simulink model "Cruise_Model_V12_CheckLin_MF"  (R2024a)
settings: Solver=VariableStepAuto  StartTime=0.0  StopTime=0.4  RelTol=1e-9
values from neighbouring files (symbols this model uses):
  coefficients =     [alexisignoringme3.mat]    (also in alexisignoringme4.mat)
  referenceGeo =     [alexisignoringme2.mat]    (also in alexisignoringme3.mat; alexisignoringme4.mat)
  sys = sysMat{i}    [createGainMat.m]    (also in testGains.m = sysMat{idx})
  Ue = [0.0166337400043 -5.79889018864e-09 -1.23056551726e-07 67.3559587388 0 1.57079632679 0 67.3557646602 0 1.57079632679 0 67.3619105721 ... (19 elements, 19x1)]    [alexisignoringme2.mat]    (also in alexisignoringme3.mat = [0.01662518914 6.61806403433e-08 9.21309449136e-07 1460.2523; alexisignoringme4.mat = [0 0 0 0 0 -1471.90874183 1.06985703496e-06 -4.11944256484e-; plotLQI_LQR_Comparison.m = Ut(:,idx(i)+1); testGains.m = U(:,idx+1))
  uref = [0.0193376442889 1.48757714448e-07 3.9703360685e-06 34.4337400406 0 1.41812999309 0 34.4385558366 0 1.41812999309 0 34.4274755705 ... (19 elements, 19x1)]    [alexisignoringme2.mat]    (also in alexisignoringme3.mat; alexisignoringme4.mat)
  Xe = [24.9700402552 0 -1.16861141766 0 0 0 1.12298779449e-07 -0.0450942805758 0.321650208764]    [alexisignoringme2.mat]    (also in alexisignoringme3.mat = [24.9726490597 0 -1.16896704065 0 0 0 -8.24889531393e-07 -0.; alexisignoringme4.mat = [24.9726490597 0 -1.16896704065 0 0 0 -8.24889531393e-07 0.0; plotLQI_LQR_Comparison.m = X(:,idx(i)+1); testGains.m = X(:,idx+1))
  Xes = [24.97004028 0 -1.16861086303 0 0 0 -5.01724449102e-07 -0.0450956248882 0.321650295301]    [alexisignoringme2.mat]    (also in alexisignoringme3.mat = [0.00351658839646 0 -9.99999599468 0 0 0 2.7327442949e-09 -4; alexisignoringme4.mat = [0 0 -1.11199998303 0 0 0 -1.38069247376e-09 1.48137256273e-; plotLQI_LQR_Comparison.m = X(:,idx(i)); selectQRfull.m = X(:,1))
  xref = [23.8431437085 -0.0286368661364 -1.0555761419 0 0 0 -3.25538675016e-06 -0.0440747284101 3.06708657292e-07]    [alexisignoringme2.mat]    (also in alexisignoringme3.mat; alexisignoringme4.mat)
undefined symbols (not defined in the file or in its folder): linsys1
libraries: shared6dof x1
settings Model: Creator=Jem  LastModifiedBy=Jem
settings OptimizationCC: ReuseModelBlockBuffer=off
settings RTWCC: GPUComputeCapability=3.5

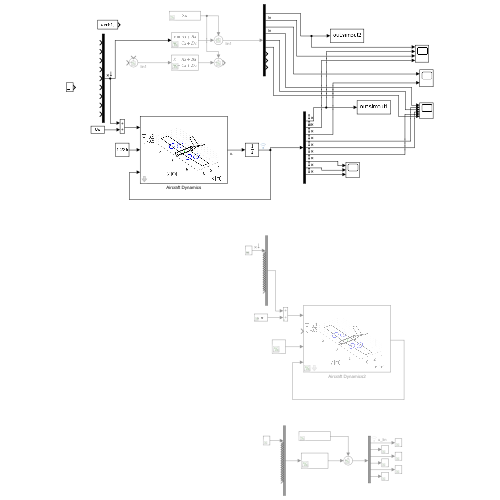
[thumbnail: Simulink's stored preview of the top-level diagram]
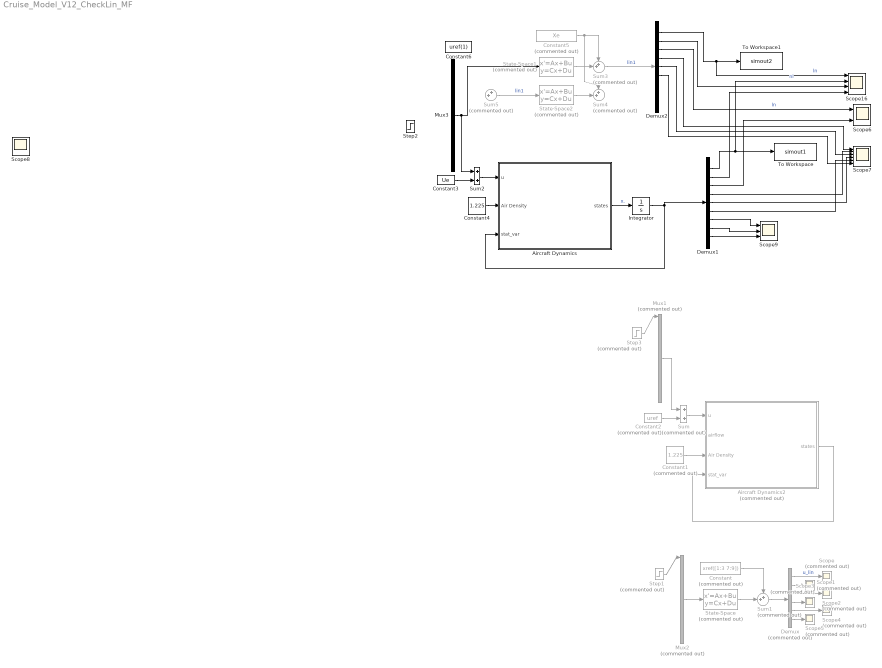
== system Cruise_Model_V12_CheckLin_MF ==
  Aircraft Dynamics : Subsystem  mask{stabDeriv_local=0, config=[], refGeo=referenceGeo, mesh=[], stabDeriv=coefficients, I=[107 0 0.6971;0 93 0;0.6971 0 196], ac=[0 0 0], cg=[1.1 0 0], m=150, uvw=Xes(1:3), lmn=Xes(7:9), pqr=Xes(4:6), xyz_e=[0 0 0], CD0=0.018, CL0=0.3, Cm0=-0.02, CDa=0.1117, CLa=3.72, CYa=0, CDb=0, CLb=0, CYb=-0.3381, Clla=0, Cma=-0.3211, Cna=0, Cllb=-0.1791, Cmb=0, Cnb=0.06724, CDn=[0 0 0], CLn=[0.1939 0 0], CYn=[0 0.02464 0.1139], Clln=[0 0.1633 -0.01337], Cmn=[0.2996 0 0], Cnn=[0 -0.01918 -0.04476], CYp=-0.09935, CYr=0.21932, CLq=4.2745, Clp=-0.3606, Clr=0.1269, Cmq=-2.708, Cnp=0.01464, Cnr=-0.04049, kt=[3.13e-05;3.13e-05;3.13e-05;3.13e-05], kb=[7.5e-07;7.5e-07;7.5e-07;7.5e-07], Tinit=[0 0 0 0], xyz_tr=[0 6.5 0.3;0 -6.5 0.3;2.2 6.5 -0.3;2.2 -6.5 -0.3], anginit=[0 0.523598775598299 0;0 0.523598775598299 0;0 0.523598775598299 0;0 0.523598775598299 0], max_def_tr=[1 -1;1 -1;1 -1;1 -1], dir=[1;-1;1;-1]}
      mask prompts: config "Configuration (object)"; refGeo "Reference Geometry (struct)"; mesh "Mesh (struct)"; stabDeriv "Stability Derivatives (struct)"; I "Inertia Tensor"; ac "Aerodynamic Centre [x y z]_ref"; cg "Centre of Gravity [x y z]_ref"; m "Mass [kg]"; uvw "[u, v, w]"; lmn "[roll, pitch, yaw]"; pqr "[p, q, r]"; xyz_e "[Xe, Ye, Ze]"; CDa "CD_a"; CLa "CL_a"; CYa "CY_a"; CDb "CD_b"; CLb "CL_b"; CYb "CY_b"; Clla "Cl_a"; Cma "Cm_a"; Cna "Cn_a"; Cllb "Cl_b"; Cmb "Cm_b"; Cnb "Cn_b"; CDn "CD_n"; CLn "CL_n"; CYn "CY_n"; Clln "Cl_n"; Cmn "Cm_n"; Cnn "Cn_n"; Tinit "Initial Thrust [kN]"; xyz_tr "XYZ_b Pos [m]"; anginit "Initial ang_b [rad]"; max_def_tr "Max [+ve -ve] Deflection (from baseline) [rad]"; dir "Rot. Dir. ([1:Clockwise, -1:Anticlockwise])"
      mask Callback config:
      | config = get_param(gcb, 'config');
      |     m = Simulink.Mask.get(gcb);
      | 
      |     if config ~= "[]"
      |     try
      |         I = evalin('base',[config '.I']);
      |         I_mask = m.getParameter('I');
      |         I_mask.Value = mat2str(I);
      | 
      |         CoL = evalin('base', [config '.CoL']);
      |         CoL_mask = m.getParameter('ac');
      |         CoL_mask.Value = mat2str(CoL);
      | 
      |         CG = evalin('base', [config '.CG']);
      |         CG_mask = m.getParameter('cg');
      |         CG_mask.Value = mat2str(CG);
      | 
      |         Cd0 = evalin('base', [config '.Cd0']);
      |         Cd0_mask = m.getParameter('CD0');
      |         Cd0_mask.Value = mat2str(Cd0);
      | 
      |         mass = evalin('base', [config '.m']);
      |         mass_mask = m.getParameter('m');
      |         mass_mask.Value = mat2str(mass);
      | 
      |         thrustObjs = evalin('base', [config '.thrust']);
      |         xyz_tr = m.getParameter('xyz_tr');
      |         anginit = m.getParameter('anginit');
      |         max_def_tr = m.getParameter('max_def_tr');
      |         Tinit = m.getParameter('Tinit');
      | 
      |         kb = m.getParameter('kb');
      |         kt = m.getParameter('kt');
      |         dir = m.getParameter('dir');
      | 
      |         xyz_tr_temp = zeros(length(thrustObjs.rotors), 3);
      |         anginit_temp = zeros(length(thrustObjs.rotors), 3);
      |         max_def_tr_temp = zeros(length(thrustObjs.rotors), 2);
      | 
      |         kb_temp = zeros(length(thrustObjs.rotors), 1);
      |         kt_temp = zeros(length(thrustObjs.rotors), 1);
      |         dir_temp = zeros(length(thrustObjs.rotors), 1);
      | 
      |         for i = 1:length(thrustObjs.rotors)
      |             xyz_tr_temp(i,1:3) = thrustObjs.rotors(i).pos;
      |             anginit_temp(i,1:3) = thrustObjs.rotors(i).ang;
      |             max_def_tr_temp(i,1:2) = thrustObjs.rotors(i).maxdef;
      | 
      |             kb_temp(i,1) = thrustObjs.rotors(i).kb;
      |             kt_temp(i,1) = thrustObjs.rotors(i).kt;
      |             dir_temp(i,1) = thrustObjs.rotors(i).dir;
      |         end
      | 
      |         xyz_tr.Value = mat2str(xyz_tr_temp);
      |         anginit.Value = mat2str(anginit_temp);
      |         max_def_tr.Value = mat2str(max_def_tr_temp);
      |         Tinit.Value = mat2str(zeros(1, length(thrustObjs.rotors)));
      | 
      |         kb.Value = mat2str(kb_temp);
      |         kt.Value = mat2str(kt_temp);
      |         dir.Value = mat2str(dir_temp);
      | 
      |         Tinit  = get_param(gcb, 'Tinit');
      |         Tinit = str2num(Tinit);
      | 
      |         n = size(Tinit,2); % number of columns
      | 
      |         load('buses.mat', "coeff", "thrust")
      | 
      |         % handled brute forcefully due to comma seperated list
      |         [thrust.Elements.Dimensions] = deal([1,n], [n,3], [n,3], [n,2]);
      | 
      |         save('buses.mat', "coeff", "thrust")
      | 
      |         disp("Configuration data extracted.")
      | 
      |     catch
      |         config = m.getParameter('config');
      |         config.Value = '[]';
      |         error('Data could not be read from specified configuration object. Please enter data manually.')
      |     end
      | 
      |     try
      |         name = get_param(gcb, 'config');
      |         config = evalin('base', name);
      |         plotConfiguration(config,0)
      | 
      |         disp("Image generated.")
      |     catch
      |         warning('Could not generate configuration image.')
      |     end
      | 
      |     end
      mask Callback stabDeriv:
      | stabDeriv = get_param(gcb, 'stabDeriv');
      |     m = Simulink.Mask.get(gcb);
      | 
      |     if stabDeriv ~= "[]"
      |         try
      |             variables = ["CL0", "Cm0", "CD0", "CLa", "CDa", "CYa", ...
      |                 "Clla", "Cma", "Cna", ...
      |                 "CLb", "CDb", "CYb", "Cllb", "Cmb", "Cnb" ...
      |                 "CDn", "CLn", "CYn", "Clln", "Cmn", "Cnn" ...
      |                 "CYp", "CYr", "CLq", "Clp", "Clr", "Cmq", "Cnp", "Cnr"];
      | 
      |             for i = 1:length(variables)
      |               param = char(variables(i));
      | 
      |               if param == "Clla"
      |                   paramws = 'Cla'; % handle case sensitivity
      |               elseif param == "Cllb"
      |                   paramws = 'Clb';
      |               elseif param == "Clln"
      |                   paramws = 'Cln';
      |               else
      |                   paramws = param;
      |               end
      | 
      |               disp(paramws)
      |               var = evalin('base',[stabDeriv '.' paramws]);
      |               var_mask = m.getParameter(param);
      |               var_mask.Value = mat2str(var);
      |               disp('here')
      |             end
      | 
      |         catch
      |           var = m.getParameter('stabDeriv');
      |           var.Value = '[]';
      |           error('Data could not be read from specified structure. Please enter data manually.')
      |         end
      | 
      |         % Handle bus sizing
      |     end
      mask Callback CLn:
      | CLn = get_param(gcb, 'CLn');
      |     n = length(str2num(CLn));
      | 
      |     load('buses.mat', "coeff", "thrust")
      | 
      |     % handled brute forcefully due to comma seperated list
      |     [coeff.Elements.Dimensions] = deal(1,1,1,1,1,1,1,1,1,1,1,1,1,1,1,n,n,n,n,n,n,1,1,1,1,1,1,1,1);
      | 
      |     save('buses.mat', "coeff", "thrust")
      |     clear coeff thrust
      mask Callback Tinit:
      | Tinit  = get_param(gcb, 'Tinit');
      |     Tinit = str2num(Tinit);
      | 
      |     n = size(Tinit,2); % number of columns
      | 
      |     load('buses.mat', "coeff", "thrust")
      | 
      |     % handled brute forcefully due to comma seperated list
      |     [thrust.Elements.Dimensions] = deal([1,n], [n,3], [n,3], [n,2], [n,1], [n,1], [n,1]);
      | 
      |     save('buses.mat', "coeff", "thrust")
      |     clear coeff thrust
      mask DialogControl ParameterGroupVar Prompt: Input Structures/Objects
      mask DialogControl Container6 Prompt: Geometry
      mask DialogControl Container4 Prompt: Initial Conditions
      mask DialogControl Container5 Prompt: Aerodynamic Derivatives
      mask DialogControl Container7 Prompt: Control Derivatives
      mask DialogControl Container8 Prompt: Coupling Derivatives
      mask DialogControl Container9 Prompt: Thrust Components
      mask Display:
      | try
      |     image('config.jpg');
      | catch
      |     image('drone.png');
      | end
  Aircraft Dynamics2 : Subsystem  Commented=on  mask{stabDeriv_local=0, config=[], refGeo=referenceGeo, mesh=[], stabDeriv=[], I=[107 0 0.6971;0 93 0;0.6971 0 196], ac=[0 0 0], cg=[1.1 0 0], m=150, uvw=xref(1:3), lmn=xref(7:9), pqr=xref(4:6), xyz_e=[0 0 0], CD0=0.018, CL0=0.3, Cm0=-0.02, CDa=0.1117, CLa=3.72, CYa=0, CDb=0, CLb=0, CYb=-0.3381, Clla=0, Cma=-0.3211, Cna=0, Cllb=-0.1791, Cmb=0, Cnb=0.06724, CDn=[0 0 0], CLn=[0.1939 0 0], CYn=[0 0.02464 0.1139], Clln=[0 0.1633 -0.01337], Cmn=[0.2996 0 0], Cnn=[0 -0.01918 -0.04476], CYp=-0.09935, CYr=0.21932, CLq=4.2745, Clp=-0.3606, Clr=0.1269, Cmq=-2.708, Cnp=0.01464, Cnr=-0.04049, Tinit=[0 0 0 0], xyz_tr=[0 3 0.3;0 -3 0.3;2.2 3 -0.3;2.2 -3 -0.3], anginit=[0 0.523598775598299 0;0 0.523598775598299 0;0 0.523598775598299 0;0 0.523598775598299 0], max_def_tr=[1 -1;1 -1;1 -1;1 -1]}
      mask prompts: config "Configuration (object)"; refGeo "Reference Geometry (struct)"; mesh "Mesh (struct)"; stabDeriv "Stability Derivatives (struct)"; I "Inertia Tensor"; ac "Aerodynamic Centre [x y z]_ref"; cg "Centre of Gravity [x y z]_ref"; m "Mass [kg]"; uvw "[u, v, w]"; lmn "[roll, pitch, yaw]"; pqr "[p, q, r]"; xyz_e "[Xe, Ye, Ze]"; CDa "CD_a"; CLa "CL_a"; CYa "CY_a"; CDb "CD_b"; CLb "CL_b"; CYb "CY_b"; Clla "Cl_a"; Cma "Cm_a"; Cna "Cn_a"; Cllb "Cl_b"; Cmb "Cm_b"; Cnb "Cn_b"; CDn "CD_n"; CLn "CL_n"; CYn "CY_n"; Clln "Cl_n"; Cmn "Cm_n"; Cnn "Cn_n"; Tinit "Initial Thrust [kN]"; xyz_tr "XYZ_b Pos [m]"; anginit "Initial ang_b [rad]"; max_def_tr "Max [+ve -ve] Deflection (from baseline) [rad]"
      mask Callback config:
      | config = get_param(gcb, 'config');
      |     m = Simulink.Mask.get(gcb);
      | 
      |     if config ~= "[]"
      |     try
      |         I = evalin('base',[config '.I']);
      |         I_mask = m.getParameter('I');
      |         I_mask.Value = mat2str(I);
      | 
      |         CoL = evalin('base', [config '.CoL']);
      |         CoL_mask = m.getParameter('ac');
      |         CoL_mask.Value = mat2str(CoL);
      | 
      |         CG = evalin('base', [config '.CG']);
      |         CG_mask = m.getParameter('cg');
      |         CG_mask.Value = mat2str(CG);
      | 
      |         Cd0 = evalin('base', [config '.Cd0']);
      |         Cd0_mask = m.getParameter('CD0');
      |         Cd0_mask.Value = mat2str(Cd0);
      | 
      |         mass = evalin('base', [config '.m']);
      |         mass_mask = m.getParameter('m');
      |         mass_mask.Value = mat2str(mass);
      | 
      |         thrustObjs = evalin('base', [config '.thrust']);
      |         xyz_tr = m.getParameter('xyz_tr');
      |         anginit = m.getParameter('anginit');
      |         max_def_tr = m.getParameter('max_def_tr');
      |         Tinit = m.getParameter('Tinit');
      | 
      |         xyz_tr_temp = zeros(length(thrustObjs.rotors), 3);
      |         anginit_temp = zeros(length(thrustObjs.rotors), 3);
      |         max_def_tr_temp = zeros(length(thrustObjs.rotors), 2);
      | 
      |         for i = 1:length(thrustObjs.rotors)
      |             xyz_tr_temp(i,1:3) = thrustObjs.rotors(i).pos;
      |             anginit_temp(i,1:3) = thrustObjs.rotors(i).ang;
      |             max_def_tr_temp(i,1:2) = thrustObjs.rotors(i).maxdef;
      |         end
      | 
      |         xyz_tr.Value = mat2str(xyz_tr_temp);
      |         anginit.Value = mat2str(anginit_temp);
      |         max_def_tr.Value = mat2str(max_def_tr_temp);
      |         Tinit.Value = mat2str(zeros(1, length(thrustObjs.rotors)));
      | 
      |         Tinit  = get_param(gcb, 'Tinit');
      |         Tinit = str2num(Tinit);
      | 
      |         n = size(Tinit,2); % number of columns
      | 
      |         load('buses.mat', "coeff", "thrust")
      | 
      |         % handled brute forcefully due to comma seperated list
      |         [thrust.Elements.Dimensions] = deal([1,n], [n,3], [n,3], [n,2]);
      | 
      |         save('buses.mat', "coeff", "thrust")
      | 
      |         disp("Configuration data extracted.")
      | 
      |     catch
      |         config = m.getParameter('config');
      |         config.Value = '[]';
      |         error('Data could not be read from specified configuration object. Please enter data manually.')
      |     end
      | 
      |     try
      |         name = get_param(gcb, 'config');
      |         config = evalin('base', name);
      |         plotConfiguration(config,0)
      | 
      |         disp("Image generated.")
      |     catch
      |         warning('Could not generate configuration image.')
      |     end
      | 
      |     end
      mask Callback stabDeriv:
      | stabDeriv = get_param(gcb, 'stabDeriv');
      |     m = Simulink.Mask.get(gcb);
      | 
      |     if stabDeriv ~= "[]"
      |         disp('here')
      |         try
      |             variables = ["CLa", "CDa", "CYa", "Cla", "Cma", "Cna", "CLb", "CDb", "CYb", "Clb", "Cmb", "Cnb"];
      |             for i = 1:length(variables)
      |               param = char(variables(i));
      | 
      |               var = evalin('base',[stabDeriv '.' param]);
      |               var_mask = m.getParameter(param);
      |               var_mask.Value = mat2str(var);
      |             end
      | 
      |         catch
      |           var = m.getParameter('stabDeriv');
      |           var.Value = '[]';
      |           error('Data could not be read from specified structure. Please enter data manually.')
      |         end
      | 
      |         % Handle bus sizing
      |     end
      mask Callback CLn:
      | CLn = get_param(gcb, 'CLn');
      |     n = length(str2num(CLn));
      | 
      |     load('buses.mat', "coeff", "thrust")
      | 
      |     % handled brute forcefully due to comma seperated list
      |     [coeff.Elements.Dimensions] = deal(1,1,1,1,1,1,1,1,1,1,1,1,1,1,1,n,n,n,n,n,n,1,1,1,1,1,1,1,1);
      | 
      |     save('buses.mat', "coeff", "thrust")
      mask Callback Tinit:
      | Tinit  = get_param(gcb, 'Tinit');
      |     Tinit = str2num(Tinit);
      | 
      |     n = size(Tinit,2); % number of columns
      | 
      |     load('buses.mat', "coeff", "thrust")
      | 
      |     % handled brute forcefully due to comma seperated list
      |     [thrust.Elements.Dimensions] = deal([1,n], [n,3], [n,3], [n,2]);
      | 
      |     save('buses.mat', "coeff", "thrust")
      mask DialogControl ParameterGroupVar Prompt: Input Structures/Objects
      mask DialogControl Container6 Prompt: Geometry
      mask DialogControl Container4 Prompt: Initial Conditions
      mask DialogControl Container5 Prompt: Aerodynamic Derivatives
      mask DialogControl Container7 Prompt: Control Derivatives
      mask DialogControl Container8 Prompt: Coupling Derivatives
      mask DialogControl Container9 Prompt: Thrust Components
      mask Display:
      | try
      |     image('config.jpg');
      | catch
      |     image('drone.png');
      | end
  Constant : Constant  Commented=on  Value=xref([1:3 7:9])
  Constant1 : Constant  Commented=on  Value=1.225
  Constant2 : Constant  Commented=on  Value=uref
  Constant3 : Constant  Value=Ue
  Constant4 : Constant  Value=1.225
  Constant5 : Constant  Commented=on  Value=Xe
  Constant6 : Constant  Value=uref(1)
  Demux : Demux  Commented=on  Outputs=6
  Demux1 : Demux  Outputs=9
  Demux2 : Demux  Outputs=9
  Integrator : Integrator  InitialCondition=Xes  IgnoreLimit=on
  Mux1 : Mux  Commented=on  Inputs=19
  Mux2 : Mux  Commented=on  Inputs=19
  Mux3 : Mux  Inputs=9
  Scope{,1..5} (6 alike) : Scope  Commented=on
  Scope16 : Scope  NumInputPorts=4
  Scope6 : Scope  NumInputPorts=2
  Scope7 : Scope  NumInputPorts=6
  Scope9 : Scope  NumInputPorts=3
  State-Space : StateSpace  Commented=on  A=sys.A  B=sys.B  C=sys.C  D=sys.D  InitialCondition=0
  State-Space1 : StateSpace  Commented=on  A=sys.A  B=sys.B  C=sys.C  D=sys.D  InitialCondition=0
  State-Space2 : StateSpace  Commented=on  A=linsys1.A  B=linsys1.B  C=linsys1.C  D=linsys1.D  InitialCondition=0
  Step1 : Step  Commented=on  After=0.05  SampleTime=0
  Step2 : Step  Time=0.1  After=300  SampleTime=0
  Step3 : Step  Commented=on  After=0.05  SampleTime=0
  Sum : Sum  Commented=on
  Sum{1,3..5} (4 alike) : Sum  Commented=on  Inputs=++|
  Sum2 : Sum
  To Workspace : ToWorkspace  VariableName=simout1  SaveFormat=Timeseries  SampleTime=-1
  To Workspace1 : ToWorkspace  VariableName=simout2  SaveFormat=Timeseries  SampleTime=-1
  Scope8 : Scope
  wires:
  Aircraft Dynamics2/1(states) -> Aircraft Dynamics2/4(stat_var)
  Step3/1 -> Mux1/1
  Sum/1 -> Aircraft Dynamics2/1(u)
  State-Space/1 -> Sum1/2
  Mux2/1 -> State-Space/1
  Sum1/1 -> Demux/1
  Constant/1 -> Sum1/1
  Demux/1 -> Scope/1  "u_lin"
  Demux/2 -> Scope1/1
  Demux/3 -> Scope2/1
  Demux/4 -> Scope3/1
  Demux/5 -> Scope4/1
  Demux/6 -> Scope5/1
  Constant1/1 -> Aircraft Dynamics2/3(Air Density)
  Step1/1 -> Mux2/1
  Constant2/1 -> Sum/2
  Mux1/1 -> Sum/1
  Aircraft Dynamics/1(states) -> Integrator/1  "x."
  Integrator/1 -> Aircraft Dynamics/3(stat_var), Demux1/1
  Constant3/1 -> Sum2/2
  Sum2/1 -> Aircraft Dynamics/1(u)
  Constant4/1 -> Aircraft Dynamics/2(Air Density)
  Demux1/1 -> Scope16/2, To Workspace/1  "nl"
  State-Space1/1 -> Sum3/2
  Constant5/1 -> Sum4/1, Sum3/1
  Mux3/1 -> Sum2/1, State-Space1/1
  State-Space2/1 -> Sum4/2
  Sum5/1 -> State-Space2/1  "lin1"
  Sum3/1 -> Demux2/1  "lin1"
  Demux2/1 -> Scope16/1, To Workspace1/1  "ln"
  Demux1/2 -> Scope16/4
  Demux1/3 -> Scope6/2
  Demux2/2 -> Scope16/3
  Demux2/3 -> Scope6/1  "ln"
  Demux2/4 -> Scope7/1
  Demux1/4 -> Scope7/2
  Demux2/5 -> Scope7/3
  Demux1/5 -> Scope7/4
  Demux2/6 -> Scope7/6
  Demux1/6 -> Scope7/5
  Demux1/7 -> Scope9/1
  Demux1/8 -> Scope9/2
  Demux1/9 -> Scope9/3

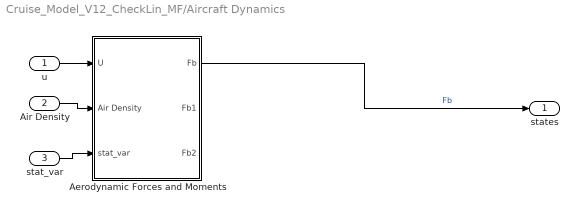
== system Cruise_Model_V12_CheckLin_MF/Aircraft Dynamics ==
  u : Inport
  Air Density : Inport  Port=2
  stat_var : Inport  Port=3
  Aerodynamic Forces and Moments : Subsystem
  states : Outport
  wires:
  u/1 -> Aerodynamic Forces and Moments/1(U)
  Air Density/1 -> Aerodynamic Forces and Moments/2(Air Density)
  stat_var/1 -> Aerodynamic Forces and Moments/3(stat_var)
  Aerodynamic Forces and Moments/1(Fb) -> states/1  "Fb"

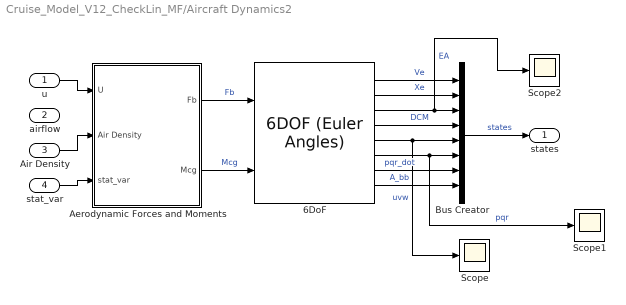
== system Cruise_Model_V12_CheckLin_MF/Aircraft Dynamics2 ==
  u : Inport
  airflow : Inport  Port=2
  Air Density : Inport  Port=3
  stat_var : Inport  Port=4
  6DoF : shared6dof/6DOF (Euler Angles)  units=Metric (MKS)  mtype=Fixed  rep=Euler Angles  xme_0=xyz_e  Vm_0=uvw  eul_0=lmn  pm_0=pqr  mass_0=m  mass_e=0.5  mass_f=2.0  inertia=I  inertia_e=eye(3)  inertia_f=2*eye(3)  k_quat=1.0  vre_flag=on  abi_flag=off  aMode=0  xme_statename=''  Vm_statename=''  eul_statename=''  quat_statename=''  pm_statename=''  mass_statename=''
  Aerodynamic Forces and Moments : Subsystem
  Bus Creator : BusCreator  Inputs=8
  Scope : Scope
  Scope1 : Scope
  Scope2 : Scope
  states : Outport
  wires:
  Aerodynamic Forces and Moments/2(Mcg) -> 6DoF/2  "Mcg"
  Aerodynamic Forces and Moments/1(Fb) -> 6DoF/1  "Fb"
  Bus Creator/1 -> states/1  "states"
  6DoF/2 -> Bus Creator/2  "Xe"
  6DoF/8 -> Bus Creator/8  "A_bb"
  6DoF/4 -> Bus Creator/4  "DCM"
  6DoF/7 -> Bus Creator/7  "pqr_dot"
  6DoF/1 -> Bus Creator/1  "Ve"
  6DoF/6 -> Scope1/1, Bus Creator/6  "pqr"
  6DoF/5 -> Bus Creator/5, Scope/1  "uvw"
  6DoF/3 -> Scope2/1, Bus Creator/3  "EA"
  u/1 -> Aerodynamic Forces and Moments/1(U)
  Air Density/1 -> Aerodynamic Forces and Moments/2(Air Density)
  stat_var/1 -> Aerodynamic Forces and Moments/3(stat_var)

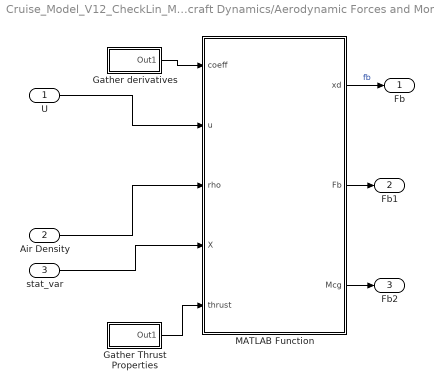
== system Cruise_Model_V12_CheckLin_MF/Aircraft Dynamics/Aerodynamic Forces and Moments ==
  U : Inport
  Air Density : Inport  Port=2
  stat_var : Inport  Port=3
  Gather Thrust Properties : Subsystem
  Gather derivatives : Subsystem
  MATLAB Function : MATLAB Function  InitFcn=load buses.mat  StartFcn=load buses.mat  TreatAsAtomicUnit=on  VariantControl=Choice  mask{refGeo=referenceGeo}
      settings: OpenFcn=load buses.mat
  Fb : Outport
  Fb1 : Outport  Port=2
  Fb2 : Outport  Port=3
  wires:
  Gather derivatives/1(Out1) -> MATLAB Function/1(coeff)
  U/1 -> MATLAB Function/2(u)
  Air Density/1 -> MATLAB Function/3(rho)
  Gather Thrust Properties/1(Out1) -> MATLAB Function/5(thrust)
  MATLAB Function/1(xd) -> Fb/1  "fb"
  stat_var/1 -> MATLAB Function/4(X)
  MATLAB Function/2(Fb) -> Fb1/1
  MATLAB Function/3(Mcg) -> Fb2/1

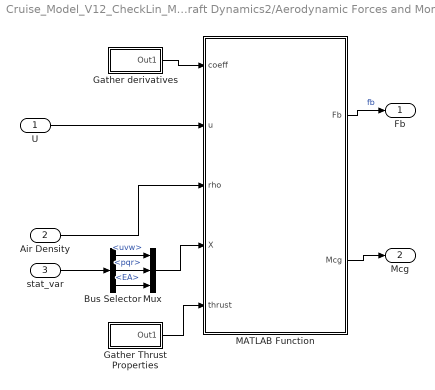
== system Cruise_Model_V12_CheckLin_MF/Aircraft Dynamics2/Aerodynamic Forces and Moments ==
  U : Inport
  Air Density : Inport  Port=2
  stat_var : Inport  Port=3
  Bus Selector : BusSelector  OutputSignals=uvw,pqr,EA
  Gather Thrust Properties : Subsystem
  Gather derivatives : Subsystem
  MATLAB Function : MATLAB Function  InitFcn=load buses.mat  StartFcn=load buses.mat  TreatAsAtomicUnit=on  VariantControl=Choice  mask{refGeo=referenceGeo}
      settings: OpenFcn=load buses.mat
  Mux : Mux  Inputs=3
  Fb : Outport
  Mcg : Outport  Port=2
  wires:
  stat_var/1 -> Bus Selector/1
  Bus Selector/1 -> Mux/1  "<uvw>"
  Bus Selector/2 -> Mux/2  "<pqr>"
  Bus Selector/3 -> Mux/3  "<EA>"
  Gather derivatives/1(Out1) -> MATLAB Function/1(coeff)
  U/1 -> MATLAB Function/2(u)
  Air Density/1 -> MATLAB Function/3(rho)
  Mux/1 -> MATLAB Function/4(X)
  Gather Thrust Properties/1(Out1) -> MATLAB Function/5(thrust)
  MATLAB Function/1(Fb) -> Fb/1  "fb"
  MATLAB Function/2(Mcg) -> Mcg/1

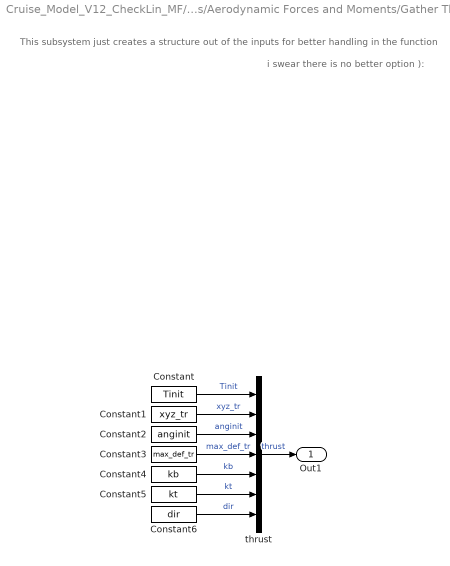
== system Cruise_Model_V12_CheckLin_MF/Aircraft Dynamics/Aerodynamic Forces and Moments/Gather Thrust Properties ==
  note: This subsystem just creates a structure out of the inputs for better handling in the function
  note: i swear there is no better option ):
  Constant : Constant  Value=Tinit
  Constant1 : Constant  Value=xyz_tr
  Constant2 : Constant  Value=anginit
  Constant3 : Constant  Value=max_def_tr
  Constant4 : Constant  Value=kb
  Constant5 : Constant  Value=kt
  Constant6 : Constant  Value=dir
  thrust : BusCreator  Inputs=7  OutDataTypeStr=Bus: thrust
  Out1 : Outport
  wires:
  thrust/1 -> Out1/1  "thrust"
  Constant/1 -> thrust/1  "Tinit"
  Constant1/1 -> thrust/2  "xyz_tr"
  Constant2/1 -> thrust/3  "anginit"
  Constant3/1 -> thrust/4  "max_def_tr"
  Constant4/1 -> thrust/5  "kb"
  Constant5/1 -> thrust/6  "kt"
  Constant6/1 -> thrust/7  "dir"

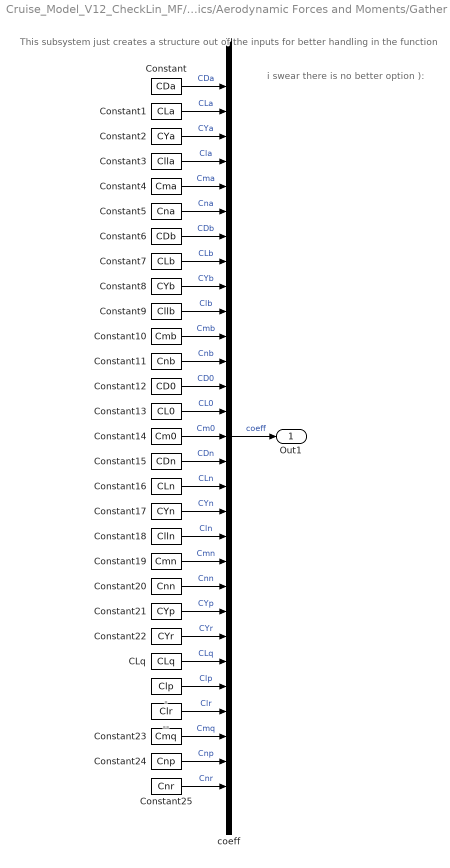
== system Cruise_Model_V12_CheckLin_MF/Aircraft Dynamics/Aerodynamic Forces and Moments/Gather derivatives ==
  note: i swear there is no better option ):
  note: This subsystem just creates a structure out of the inputs for better handling in the function
  - : Constant  Value=Clp
  -- : Constant  Value=Clr
  CLq : Constant  Value=CLq
  Constant : Constant  Value=CDa
  Constant1 : Constant  Value=CLa
  Constant10 : Constant  Value=Cmb
  Constant11 : Constant  Value=Cnb  VectorParams1D=off
  Constant12 : Constant  Value=CD0
  Constant13 : Constant  Value=CL0
  Constant14 : Constant  Value=Cm0
  Constant15 : Constant  Value=CDn
  Constant16 : Constant  Value=CLn
  Constant17 : Constant  Value=CYn
  Constant18 : Constant  Value=Clln
  Constant19 : Constant  Value=Cmn
  Constant2 : Constant  Value=CYa
  Constant20 : Constant  Value=Cnn
  Constant21 : Constant  Value=CYp
  Constant22 : Constant  Value=CYr
  Constant23 : Constant  Value=Cmq
  Constant24 : Constant  Value=Cnp
  Constant25 : Constant  Value=Cnr
  Constant3 : Constant  Value=Clla
  Constant4 : Constant  Value=Cma
  Constant5 : Constant  Value=Cna
  Constant6 : Constant  Value=CDb
  Constant7 : Constant  Value=CLb
  Constant8 : Constant  Value=CYb
  Constant9 : Constant  Value=Cllb
  coeff : BusCreator  Inputs=29
  Out1 : Outport
  wires:
  coeff/1 -> Out1/1  "coeff"
  Constant/1 -> coeff/1  "CDa"
  Constant1/1 -> coeff/2  "CLa"
  Constant2/1 -> coeff/3  "CYa"
  Constant3/1 -> coeff/4  "Cla"
  Constant4/1 -> coeff/5  "Cma"
  Constant5/1 -> coeff/6  "Cna"
  Constant11/1 -> coeff/12  "Cnb"
  Constant10/1 -> coeff/11  "Cmb"
  Constant9/1 -> coeff/10  "Clb"
  Constant8/1 -> coeff/9  "CYb"
  Constant7/1 -> coeff/8  "CLb"
  Constant6/1 -> coeff/7  "CDb"
  Constant12/1 -> coeff/13  "CD0"
  Constant13/1 -> coeff/14  "CL0"
  Constant14/1 -> coeff/15  "Cm0"
  Constant15/1 -> coeff/16  "CDn"
  Constant16/1 -> coeff/17  "CLn"
  Constant17/1 -> coeff/18  "CYn"
  Constant18/1 -> coeff/19  "Cln"
  Constant19/1 -> coeff/20  "Cmn"
  Constant20/1 -> coeff/21  "Cnn"
  Constant21/1 -> coeff/22  "CYp"
  Constant22/1 -> coeff/23  "CYr"
  CLq/1 -> coeff/24  "CLq"
  -/1 -> coeff/25  "Clp"
  --/1 -> coeff/26  "Clr"
  Constant23/1 -> coeff/27  "Cmq"
  Constant24/1 -> coeff/28  "Cnp"
  Constant25/1 -> coeff/29  "Cnr"

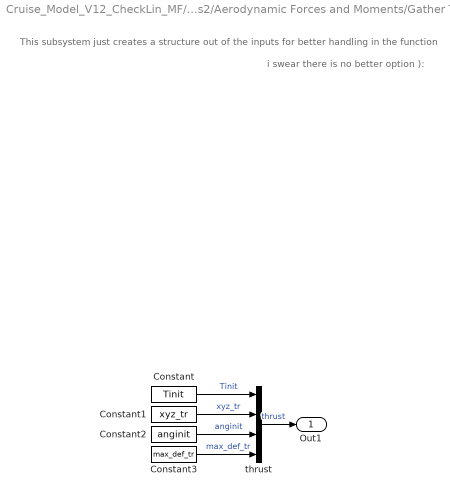
== system Cruise_Model_V12_CheckLin_MF/Aircraft Dynamics2/Aerodynamic Forces and Moments/Gather Thrust Properties ==
  note: This subsystem just creates a structure out of the inputs for better handling in the function
  note: i swear there is no better option ):
  Constant : Constant  Value=Tinit
  Constant1 : Constant  Value=xyz_tr
  Constant2 : Constant  Value=anginit
  Constant3 : Constant  Value=max_def_tr
  thrust : BusCreator  Inputs=4  OutDataTypeStr=Bus: thrust
  Out1 : Outport
  wires:
  thrust/1 -> Out1/1  "thrust"
  Constant/1 -> thrust/1  "Tinit"
  Constant1/1 -> thrust/2  "xyz_tr"
  Constant2/1 -> thrust/3  "anginit"
  Constant3/1 -> thrust/4  "max_def_tr"

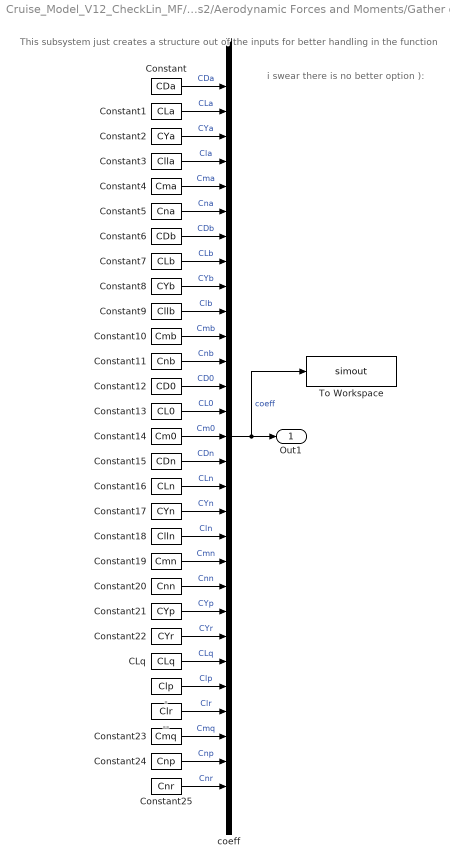
== system Cruise_Model_V12_CheckLin_MF/Aircraft Dynamics2/Aerodynamic Forces and Moments/Gather derivatives ==
  note: i swear there is no better option ):
  note: This subsystem just creates a structure out of the inputs for better handling in the function
  - : Constant  Value=Clp
  -- : Constant  Value=Clr
  CLq : Constant  Value=CLq
  Constant : Constant  Value=CDa
  Constant1 : Constant  Value=CLa
  Constant10 : Constant  Value=Cmb
  Constant11 : Constant  Value=Cnb  VectorParams1D=off
  Constant12 : Constant  Value=CD0
  Constant13 : Constant  Value=CL0
  Constant14 : Constant  Value=Cm0
  Constant15 : Constant  Value=CDn
  Constant16 : Constant  Value=CLn
  Constant17 : Constant  Value=CYn
  Constant18 : Constant  Value=Clln
  Constant19 : Constant  Value=Cmn
  Constant2 : Constant  Value=CYa
  Constant20 : Constant  Value=Cnn
  Constant21 : Constant  Value=CYp
  Constant22 : Constant  Value=CYr
  Constant23 : Constant  Value=Cmq
  Constant24 : Constant  Value=Cnp
  Constant25 : Constant  Value=Cnr
  Constant3 : Constant  Value=Clla
  Constant4 : Constant  Value=Cma
  Constant5 : Constant  Value=Cna
  Constant6 : Constant  Value=CDb
  Constant7 : Constant  Value=CLb
  Constant8 : Constant  Value=CYb
  Constant9 : Constant  Value=Cllb
  To Workspace : ToWorkspace  VariableName=simout  SaveFormat=Timeseries  SampleTime=-1
  coeff : BusCreator  Inputs=29
  Out1 : Outport
  wires:
  coeff/1 -> To Workspace/1, Out1/1  "coeff"
  Constant/1 -> coeff/1  "CDa"
  Constant1/1 -> coeff/2  "CLa"
  Constant2/1 -> coeff/3  "CYa"
  Constant3/1 -> coeff/4  "Cla"
  Constant4/1 -> coeff/5  "Cma"
  Constant5/1 -> coeff/6  "Cna"
  Constant11/1 -> coeff/12  "Cnb"
  Constant10/1 -> coeff/11  "Cmb"
  Constant9/1 -> coeff/10  "Clb"
  Constant8/1 -> coeff/9  "CYb"
  Constant7/1 -> coeff/8  "CLb"
  Constant6/1 -> coeff/7  "CDb"
  Constant12/1 -> coeff/13  "CD0"
  Constant13/1 -> coeff/14  "CL0"
  Constant14/1 -> coeff/15  "Cm0"
  Constant15/1 -> coeff/16  "CDn"
  Constant16/1 -> coeff/17  "CLn"
  Constant17/1 -> coeff/18  "CYn"
  Constant18/1 -> coeff/19  "Cln"
  Constant19/1 -> coeff/20  "Cmn"
  Constant20/1 -> coeff/21  "Cnn"
  Constant21/1 -> coeff/22  "CYp"
  Constant22/1 -> coeff/23  "CYr"
  CLq/1 -> coeff/24  "CLq"
  -/1 -> coeff/25  "Clp"
  --/1 -> coeff/26  "Clr"
  Constant23/1 -> coeff/27  "Cmq"
  Constant24/1 -> coeff/28  "Cnp"
  Constant25/1 -> coeff/29  "Cnr"

== matlab function Cruise_Model_V12_CheckLin_MF/Aircraft Dynamics/Aerodynamic Forces and Moments/MATLAB Function ==
  data: xd output; coeff input Bus: coeff; u input; rho input; X input; refGeo parameter; m parameter; thrust input; cg parameter; I parameter; Fb output; Mcg output
function [xd, Fb, Mcg]  = aeroDyn(coeff, u, rho, X, refGeo, m, thrust, cg, I)
% Function aeroDyn simulates .... Independent version (i.e. doesn't need alpha/beta/V inputs)

%% Calculate Airflow
V = sqrt(X(1)^2 + X(2)^2 + X(3)^2);
alpha = atan2(X(3), X(1));
beta = atan2(X(2), X(1));

%% Setting up intermediate variables
b = refGeo.bref;
S = refGeo.Sref;
c = refGeo.cref;

Q = 0.5*rho*V^2; % Dynamic pressure Q

ndc = c/(2*V);
ndb = b/(2*V);

%% Seperating vectors (BFR)
uvw = X(1:3); % Translational velocity vector
pqr = X(4:6); % Angular velocity vector
EA = X(7:end);

%% Handle Stall

%% Non-dimensional Aerodynamic Force Coefficients
% In wind axis
% Lift
CL = applyDeriv(coeff.CL0, coeff.CLa, coeff.CLb, coeff.CLn, 0, coeff.CLq, 0, u, alpha, beta, pqr, ndc);

% Drag 
CD = applyDeriv(coeff.CD0, coeff.CDa, coeff.CDb, coeff.CDn, 0, 0, 0, u, abs(alpha), beta, pqr, ndc);

% Sideforce
CY = applyDeriv(0, coeff.CYa, coeff.CYb, coeff.CYn, coeff.CYp, 0, coeff.CYr, u, alpha, beta, pqr, ndb);

if abs(alpha) > 14.5*(pi/180)
    CL = 0;
    CD = coeff.CD0;
end

%% Rotate wind to body
Faw = [-max(CD,0); CY; -CL].*Q*S; % Force vector in the stability frame

Rwb = [cos(alpha)*cos(beta), -cos(alpha)*sin(beta), -sin(alpha);  
       sin(beta)           ,  cos(beta)           ,  0         ; 
       cos(beta)*sin(alpha), -sin(alpha)*sin(beta),  cos(alpha)];

Fab = Rwb*Faw; % aerodynamic force on body

%% Aerodynamic Moment about CG
% In Fb, with moments taken about the centre of gravity

% Roll
Cl = applyDeriv(0, coeff.Cla, coeff.Clb, coeff.Cln, coeff.Clp, 0, coeff.Clr, u, alpha, beta, pqr, ndb);

% Pitch
Cm = applyDeriv(coeff.Cm0, coeff.Cma, coeff.Cmb, coeff.Cmn, 0, coeff.Cmq, 0, u, alpha, beta, pqr, ndc);

% Yaw
Cn = applyDeriv(0, coeff.Cna, coeff.Cnb, coeff.Cnn, coeff.Cnp, 0, coeff.Cnr, u, alpha, beta, pqr, ndb);

if abs(alpha) > 14.5*(pi/180)
    Cm = 0;
end

Ma = [b*Cl; c*Cm; b*Cn].*Q*S;

%% Propulsion Effects
% Moment and forces induced by throttle
FTb = u(4:6);
MTcg = u(7:9);

% Gravity Effects
Fgb = [-9.81*sin(X(8))          ; % Body frame
        9.81*cos(X(8))*sin(X(7));
        9.81*cos(X(8))*cos(X(7))]*m; % ASSUMPTION: Constant Mass

%% Out
Rbe = body2earth(X(7), X(8), X(9));

Fb = FTb + Fgb + Fab;
Mcg = MTcg + Ma;

forces = [FTb; Fgb; Fab; Rbe*Fb];
aero = [CL; CD; Cm];
uvw_e = Rbe*X(1:3);

xd = explicitFO(Fb, Mcg, I, X, m)';

end

%% Extra functions

function C = applyDeriv(C0, Ca, Cb, Cn, Cp, Cq, Cr, u, alpha, beta, pqr, nd)
% function applyDeriv calculates the coefficient C from the derivatives C0,
% Ca, Cb, Cn wrt 0, alpha, beta and control (n), respectively.

    C_nc = C0 + Ca*alpha + Cb*beta + Cp*pqr(1)*nd + Cq*pqr(2)*nd + Cr*pqr(3)*nd; % lift coefficient no control
    
    C_c = (Cn.*u(1:length(Cn)))';

    C = C_nc + sum(C_c);

end

== matlab function Cruise_Model_V12_CheckLin_MF/Aircraft Dynamics2/Aerodynamic Forces and Moments/MATLAB Function ==
  data: Fb output; Mcg output; coeff input Bus: coeff; u input; rho input; X input; refGeo parameter; m parameter; thrust input; cg parameter
function [Fb,Mcg] = aeroDyn(coeff, u, rho, X, refGeo, m, thrust, cg)
% Function aeroDyn simulates ....

%% Calculate Airflow
V = sqrt(X(1)^2 + X(2)^2 + X(3)^2);
alpha = atan2(X(3), X(1));
beta = atan2(X(2), X(1));

%% Setting up intermediate variables
b = refGeo.bref;
S = refGeo.Sref;
c = refGeo.cref;

Q = 0.5*rho*V^2; % Dynamic pressure Q

ndc = c/(2*V);
ndb = b/(2*V);

%% Seperating vectors (BFR)
uvw = X(1:3); % Translational velocity vector
pqr = X(4:6); % Angular velocity vector
EA = X(7:end);

%% Handle Stall

%% Non-dimensional Aerodynamic Force Coefficients
% In wind axis
% Lift
CL = applyDeriv(coeff.CL0, coeff.CLa, coeff.CLb, coeff.CLn, 0, coeff.CLq, 0, u, alpha, beta, pqr, ndc);

% Drag 
CD = applyDeriv(coeff.CD0, coeff.CDa, coeff.CDb, coeff.CDn, 0, 0, 0, u, alpha, beta, pqr, ndc);

% Sideforce
CY = applyDeriv(0, coeff.CYa, coeff.CYb, coeff.CYn, coeff.CYp, 0, coeff.CYr, u, alpha, beta, pqr, ndb);

if abs(alpha) > 20*(pi/180)
    CL = 0;
end

%% Rotate wind to body
Faw = [-max(CD,0); CY; -CL].*Q*S; % Force vector in the stability frame

Rwb = [cos(alpha)*cos(beta), -cos(alpha)*sin(beta), -sin(alpha);  
       sin(beta)           ,  cos(beta)           ,  0         ; 
       cos(beta)*sin(alpha), -sin(alpha)*sin(beta),  cos(alpha)];

Fab = Rwb*Faw; % aerodynamic force on body

%% Aerodynamic Moment about CG
% In Fb, with moments taken about the centre of gravity

% Roll
Cl = applyDeriv(0, coeff.Cla, coeff.Clb, coeff.Cln, coeff.Clp, 0, coeff.Clr, u, alpha, beta, pqr, ndb);

% Pitch
Cm = applyDeriv(coeff.Cm0, coeff.Cma, coeff.Cmb, coeff.Cmn, 0, coeff.Cmq, 0, u, alpha, beta, pqr, ndc);

% Yaw
Cn = applyDeriv(0, coeff.Cna, coeff.Cnb, coeff.Cnn, coeff.Cnp, 0, coeff.Cnr, u, alpha, beta, pqr, ndb);

if abs(alpha) > 20*(pi/180)
    Cm = 0;
end

Ma = [b*Cl; c*Cm; b*Cn].*Q*S;

%% Propulsion Effects
% Moment and forces induced by throttle
FTb = zeros(3, length(thrust.Tinit));
MTcg = zeros(3, length(thrust.Tinit));

for i = 1:length(thrust.Tinit)
    idx = length(coeff.CLn) + 1 + (i-1)*4; % index of thrust-deflection pairs for thrust objects
    FTt = [0      ; % Thrust in rotor plane
           0      ;
           -u(idx)];
    
    Rrb = transMatrix([u(idx+1) u(idx+2) u(idx+3)].*[1 1 1]); % rotation matrix from rotor plane to body, first converting to geometric axis

    FTb(:,i) = Rrb*FTt; % Rotate to body frame, switching from geometric to dynamic coordinates
    MTcg(:,i) = cross(thrust.xyz_tr(i,:) - cg, FTb(:,i));
end

FTb = sum(FTb,2);
MTcg = sum(MTcg,2);

% Gravity Effects
Fgb = [-9.81*sin(X(8))          ; % Body frame
        9.81*cos(X(8))*sin(X(7));
        9.81*cos(X(8))*cos(X(7))]*m; % ASSUMPTION: Constant Mass

%% Out
Fb = FTb + Fgb + Fab;
Mcg = MTcg + Ma;

end

%% Extra functions

function C = applyDeriv(C0, Ca, Cb, Cn, Cp, Cq, Cr, u, alpha, beta, pqr, nd)
% function applyDeriv calculates the coefficient C from the derivatives C0,
% Ca, Cb, Cn wrt 0, alpha, beta and control (n), respectively.

    C_nc = C0 + Ca*alpha + Cb*beta + Cp*pqr(1)*nd + Cq*pqr(2)*nd + Cr*pqr(3)*nd; % lift coefficient no control
    
    C_c = (Cn.*u(1:length(Cn)))';

    C = C_nc + sum(C_c);

end
